simulink subsystem "GeneratorGam_ref_SubSystem"  (R2020b)
settings: Solver=VariableStepAuto  StartTime=0.0  StopTime=10.0  RelTol=1e-3
undefined symbols (not defined in the file): enable_Ref_Tracking, Ts, wheel
settings Model: Creator=umberto  LastModifiedBy=Musta

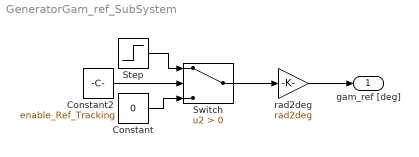
== system GeneratorGam_ref_SubSystem ==
  Constant : Constant  Value=0  SampleTime=Ts
  Constant2 : Constant  Value=enable_Ref_Tracking
  Step : Step  Time=10  After=0.1/wheel.r  SampleTime=Ts
  Switch : Switch  Criteria=u2 > Threshold
  rad2deg : Gain  Gain=rad2deg
  gam_ref [deg] : Outport
  wires:
  rad2deg/1 -> gam_ref [deg]/1
  Switch/1 -> rad2deg/1
  Step/1 -> Switch/1
  Constant2/1 -> Switch/2
  Constant/1 -> Switch/3
